simulink library "FUSI"  (R2024b)
settings: Solver=VariableStepAuto  StartTime=0.0  StopTime=10.0  RelTol=1e-3
libraries: simulink x1, FUSA_ACTMON x1, FUSA_FAULTVAIMAN x1, FUSA_SENSMON x1
settings Model: Creator=blatak  LastModifiedBy=jmbsp
settings ModelReferenceCC: EnableRefExpFcnMdlSchedulingChecks=on
settings RTWCC: GPUComputeCapability=3.5

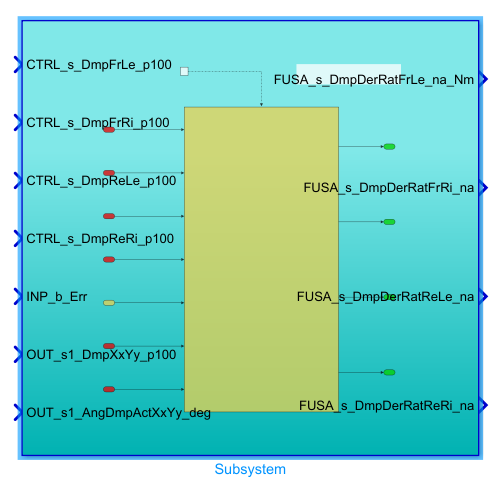
[thumbnail: Simulink's stored preview of the top-level diagram]
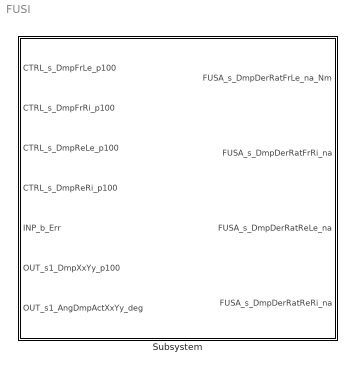
== system FUSI ==
  Subsystem : Subsystem

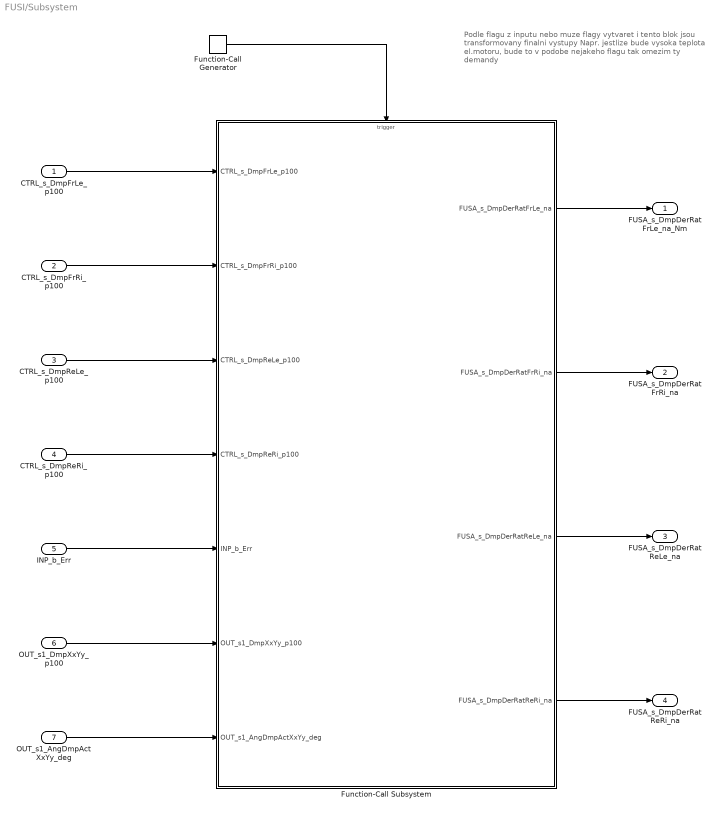
== system FUSI/Subsystem ==
  note: Podle flagu z inputu nebo muze flagy vytvaret i tento blok
      | jsou transformovany finalni vystupy
      | Napr. jestlize bude vysoka teplota el.motoru, bude to v podobe
      | nejakeho flagu tak omezim ty demandy
  CTRL_s_DmpFrLe_p100 : Inport
  CTRL_s_DmpFrRi_p100 : Inport  Port=2
  CTRL_s_DmpReLe_p100 : Inport  Port=3
  CTRL_s_DmpReRi_p100 : Inport  Port=4
  INP_b_Err : Inport  Port=5  OutDataTypeStr=Bus: INP_b_Err
  OUT_s1_DmpXxYy_p100 : Inport  Port=6
  OUT_s1_AngDmpActXxYy_deg : Inport  Port=7
  Function-Call Generator : simulink/Ports & Subsystems/Function-Call Generator  sample_time=0.005  numberOfIterations=1  DisallowWideOutput=off
  Function-Call Subsystem : Subsystem  TreatAsAtomicUnit=on
  FUSA_s_DmpDerRatFrLe_na_Nm : Outport
  FUSA_s_DmpDerRatFrRi_na : Outport  Port=2
  FUSA_s_DmpDerRatReLe_na : Outport  Port=3
  FUSA_s_DmpDerRatReRi_na : Outport  Port=4
  wires:
  Function-Call Generator/1 -> Function-Call Subsystem/Trigger
  CTRL_s_DmpFrLe_p100/1 -> Function-Call Subsystem/1(CTRL_s_DmpFrLe_p100)
  CTRL_s_DmpFrRi_p100/1 -> Function-Call Subsystem/2(CTRL_s_DmpFrRi_p100)
  CTRL_s_DmpReLe_p100/1 -> Function-Call Subsystem/3(CTRL_s_DmpReLe_p100)
  CTRL_s_DmpReRi_p100/1 -> Function-Call Subsystem/4(CTRL_s_DmpReRi_p100)
  Function-Call Subsystem/1(FUSA_s_DmpDerRatFrLe_na) -> FUSA_s_DmpDerRatFrLe_na_Nm/1
  INP_b_Err/1 -> Function-Call Subsystem/5(INP_b_Err)
  Function-Call Subsystem/2(FUSA_s_DmpDerRatFrRi_na) -> FUSA_s_DmpDerRatFrRi_na/1
  Function-Call Subsystem/3(FUSA_s_DmpDerRatReLe_na) -> FUSA_s_DmpDerRatReLe_na/1
  Function-Call Subsystem/4(FUSA_s_DmpDerRatReRi_na) -> FUSA_s_DmpDerRatReRi_na/1
  OUT_s1_DmpXxYy_p100/1 -> Function-Call Subsystem/6(OUT_s1_DmpXxYy_p100)
  OUT_s1_AngDmpActXxYy_deg/1 -> Function-Call Subsystem/7(OUT_s1_AngDmpActXxYy_deg)

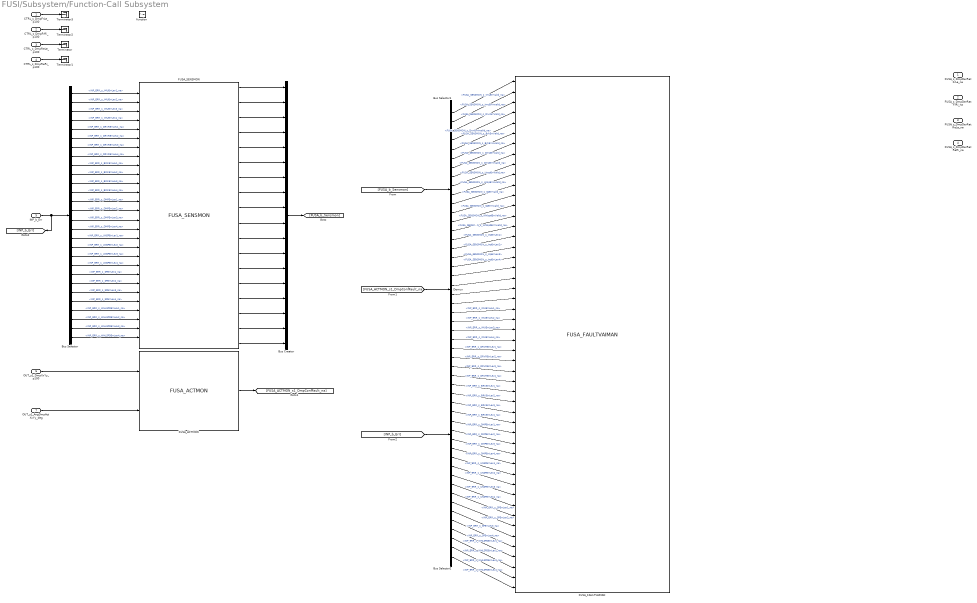
== system FUSI/Subsystem/Function-Call Subsystem ==
  CTRL_s_DmpFrLe_p100 : Inport
  CTRL_s_DmpFrRi_p100 : Inport  Port=2
  CTRL_s_DmpReLe_p100 : Inport  Port=3
  CTRL_s_DmpReRi_p100 : Inport  Port=4
  INP_b_Err : Inport  Port=5  OutDataTypeStr=Bus: INP_b_Err
  OUT_s1_DmpXxYy_p100 : Inport  Port=6
  OUT_s1_AngDmpActXxYy_deg : Inport  Port=7
  function : TriggerPort  TriggerType=function-call  VariantControl=(inherit)
  Bus Creator : BusCreator  Inputs=18  OutDataTypeStr=Bus: FUSA_b_Sensmon
      settings: InheritFromInputs=off
  Bus Selector : BusSelector  OutputSignals=INP_ERR_s_IMUErrLev1_na,INP_ERR_s_IMUErrLev2_na,INP_ERR_s_IMUErrLev3_na,INP_ERR_s_IMUErrLev4_na,INP_ERR_s_DRVRErrLev1_na,INP_ERR_s_DRVRErrLev2_na,INP_ERR_s_DRVRErrLev3_na,INP_ERR_s_DRVRErrLev4_na,INP_ERR_s_BRKErrLev1_na,INP_ERR_s_BRKErrLev2_na,INP_ERR_s_BRKErrLev3_na,INP_ERR_s_BRKErrLev4_na,INP_ERR_s_DMPErrLev1_na,INP_ERR_s_DMPErrLev2_na,INP_ERR_s_DMPErrLev3_na,INP_ERR_s_DMPErrLev4_na,INP_ERR_s_UNSPErrLev1_na,INP_ERR_s_UNSPErrLev2_na,INP_ERR_s_UNSPErrLev3_na,INP_ERR_s_UNSPErrLev4_na,INP_ERR_s_SPErrLev1_na,INP_ERR_s_SPErrLev2_na,INP_ERR_s_SPErrLev3_na,INP_ERR_s_SPErrLev4_na,INP_ERR_s_WHLSPDErrLev1_na,INP_ERR_s_WHLSPDErrLev2_na,INP_ERR_s_WHLSPDErrLev3_na,INP_ERR_s_WHLSPDErrLev4_na
  Bus Selector1 : BusSelector  OutputSignals=FUSA_SENSMON_s_ImuErrValid_na,FUSA_SENSMON_s_ImuErrInvalid_na,FUSA_SENSMON_s_DrvrErrValid_na,FUSA_SENSMON_s_DrvrErrInvalid_na,FUSA_SENSMON_s_BrkErrValid_na,FUSA_SENSMON_s_BrkErrInvalid_na,FUSA_SENSMON_s_DmpErrValid_na,FUSA_SENSMON_s_DmpErrInvalid_na,FUSA_SENSMON_s_UnspErrValid_na,FUSA_SENSMON_s_UnspErrInvalid_na,FUSA_SENSMON_s_SpErrValid_na,FUSA_SENSMON_s_SpErrInvalid_na,FUSA_SENSMON_s_WhlspdErrValid_na,FUSA_SENSMON_s_WhlspdErrInvalid_na,FUSA_SENSMON_s_InpErrLev1,FUSA_SENSMON_s_InpErrLev2,FUSA_SENSMON_s_InpErrLev3,FUSA_SENSMON_s_InpErrLev4
  Bus Selector2 : BusSelector  OutputSignals=INP_ERR_s_IMUErrLev1_na,INP_ERR_s_IMUErrLev2_na,INP_ERR_s_IMUErrLev3_na,INP_ERR_s_IMUErrLev4_na,INP_ERR_s_DRVRErrLev1_na,INP_ERR_s_DRVRErrLev2_na,INP_ERR_s_DRVRErrLev3_na,INP_ERR_s_DRVRErrLev4_na,INP_ERR_s_BRKErrLev1_na,INP_ERR_s_BRKErrLev2_na,INP_ERR_s_BRKErrLev3_na,INP_ERR_s_BRKErrLev4_na,INP_ERR_s_DMPErrLev1_na,INP_ERR_s_DMPErrLev2_na,INP_ERR_s_DMPErrLev3_na,INP_ERR_s_DMPErrLev4_na,INP_ERR_s_UNSPErrLev1_na,INP_ERR_s_UNSPErrLev2_na,INP_ERR_s_UNSPErrLev3_na,INP_ERR_s_UNSPErrLev4_na,INP_ERR_s_SPErrLev1_na,INP_ERR_s_SPErrLev2_na,INP_ERR_s_SPErrLev3_na,INP_ERR_s_SPErrLev4_na,INP_ERR_s_WHLSPDErrLev1_na,INP_ERR_s_WHLSPDErrLev2_na,INP_ERR_s_WHLSPDErrLev3_na,INP_ERR_s_WHLSPDErrLev4_na
  Demux : Demux
  FUSA_ACTMON : FUSA_ACTMON/FUSA_ACTMON  SystemSampleTime=-1  VariantActivationTime=update diagram  AllowFlexibleInterface=on  Latency=0  AutoFrameSizeCalculation=off
  FUSA_FAULTVAIMAN : FUSA_FAULTVAIMAN/FUSA_FAULTVAIMAN  SystemSampleTime=-1  VariantActivationTime=update diagram  AllowFlexibleInterface=on  Latency=0  AutoFrameSizeCalculation=off
  FUSA_SENSMON : FUSA_SENSMON/FUSA_SENSMON  SystemSampleTime=-1  VariantActivationTime=update diagram  AllowFlexibleInterface=on  Latency=0  AutoFrameSizeCalculation=off
  Terminator{,1..3} (4 alike) : Terminator
  FUSA_s_DmpDerRatFrLe_na : Outport
  FUSA_s_DmpDerRatFrRi_na : Outport  Port=2
  FUSA_s_DmpDerRatReLe_na : Outport  Port=3
  FUSA_s_DmpDerRatReRi_na : Outport  Port=4
  wires:
  INP_b_Err/1 -> [INP_b_Err], Bus Selector/1
  OUT_s1_DmpXxYy_p100/1 -> FUSA_ACTMON/1
  OUT_s1_AngDmpActXxYy_deg/1 -> FUSA_ACTMON/2
  Bus Selector/23 -> FUSA_SENSMON/23  "<INP_ERR_s_SPErrLev3_na>"
  Bus Selector/24 -> FUSA_SENSMON/24  "<INP_ERR_s_SPErrLev4_na>"
  Bus Selector/22 -> FUSA_SENSMON/22  "<INP_ERR_s_SPErrLev2_na>"
  Bus Selector/25 -> FUSA_SENSMON/25  "<INP_ERR_s_WHLSPDErrLev1_na>"
  Bus Selector/21 -> FUSA_SENSMON/21  "<INP_ERR_s_SPErrLev1_na>"
  Bus Selector/26 -> FUSA_SENSMON/26  "<INP_ERR_s_WHLSPDErrLev2_na>"
  Bus Selector/20 -> FUSA_SENSMON/20  "<INP_ERR_s_UNSPErrLev4_na>"
  Bus Selector/27 -> FUSA_SENSMON/27  "<INP_ERR_s_WHLSPDErrLev3_na>"
  Bus Selector/19 -> FUSA_SENSMON/19  "<INP_ERR_s_UNSPErrLev3_na>"
  Bus Selector/28 -> FUSA_SENSMON/28  "<INP_ERR_s_WHLSPDErrLev4_na>"
  Bus Selector/18 -> FUSA_SENSMON/18  "<INP_ERR_s_UNSPErrLev2_na>"
  Bus Selector/17 -> FUSA_SENSMON/17  "<INP_ERR_s_UNSPErrLev1_na>"
  Bus Selector/16 -> FUSA_SENSMON/16  "<INP_ERR_s_DMPErrLev4_na>"
  Bus Selector/15 -> FUSA_SENSMON/15  "<INP_ERR_s_DMPErrLev3_na>"
  Bus Selector/14 -> FUSA_SENSMON/14  "<INP_ERR_s_DMPErrLev2_na>"
  Bus Selector/13 -> FUSA_SENSMON/13  "<INP_ERR_s_DMPErrLev1_na>"
  Bus Selector/12 -> FUSA_SENSMON/12  "<INP_ERR_s_BRKErrLev4_na>"
  Bus Selector/11 -> FUSA_SENSMON/11  "<INP_ERR_s_BRKErrLev3_na>"
  Bus Selector/10 -> FUSA_SENSMON/10  "<INP_ERR_s_BRKErrLev2_na>"
  Bus Selector/9 -> FUSA_SENSMON/9  "<INP_ERR_s_BRKErrLev1_na>"
  Bus Selector/8 -> FUSA_SENSMON/8  "<INP_ERR_s_DRVRErrLev4_na>"
  Bus Selector/7 -> FUSA_SENSMON/7  "<INP_ERR_s_DRVRErrLev3_na>"
  Bus Selector/6 -> FUSA_SENSMON/6  "<INP_ERR_s_DRVRErrLev2_na>"
  Bus Selector/5 -> FUSA_SENSMON/5  "<INP_ERR_s_DRVRErrLev1_na>"
  Bus Selector/4 -> FUSA_SENSMON/4  "<INP_ERR_s_IMUErrLev4_na>"
  Bus Selector/3 -> FUSA_SENSMON/3  "<INP_ERR_s_IMUErrLev3_na>"
  Bus Selector/2 -> FUSA_SENSMON/2  "<INP_ERR_s_IMUErrLev2_na>"
  Bus Selector/1 -> FUSA_SENSMON/1  "<INP_ERR_s_IMUErrLev1_na>"
  FUSA_SENSMON/1 -> Bus Creator/1
  FUSA_SENSMON/2 -> Bus Creator/2
  FUSA_SENSMON/3 -> Bus Creator/3
  FUSA_SENSMON/4 -> Bus Creator/4
  FUSA_SENSMON/5 -> Bus Creator/5
  FUSA_SENSMON/6 -> Bus Creator/6
  FUSA_SENSMON/7 -> Bus Creator/7
  FUSA_SENSMON/8 -> Bus Creator/8
  FUSA_SENSMON/9 -> Bus Creator/9
  FUSA_SENSMON/10 -> Bus Creator/10
  FUSA_SENSMON/11 -> Bus Creator/11
  FUSA_SENSMON/12 -> Bus Creator/12
  FUSA_SENSMON/13 -> Bus Creator/13
  FUSA_SENSMON/14 -> Bus Creator/14
  FUSA_SENSMON/15 -> Bus Creator/15
  FUSA_SENSMON/16 -> Bus Creator/16
  FUSA_SENSMON/17 -> Bus Creator/17
  FUSA_SENSMON/18 -> Bus Creator/18
  Bus Creator/1 -> [FUSA_b_Sensmon]
  CTRL_s_DmpReLe_p100/1 -> Terminator/1
  CTRL_s_DmpReRi_p100/1 -> Terminator1/1
  CTRL_s_DmpFrRi_p100/1 -> Terminator2/1
  CTRL_s_DmpFrLe_p100/1 -> Terminator3/1
  FUSA_ACTMON/1 -> [FUSA_ACTMON_s1_DmpConfFault_na]
  [FUSA_ACTMON_s1_DmpConfFault_na] -> Demux/1
  [FUSA_b_Sensmon] -> Bus Selector1/1
  Bus Selector1/1 -> FUSA_FAULTVAIMAN/1  "<FUSA_SENSMON_s_ImuErrValid_na>"
  Bus Selector1/2 -> FUSA_FAULTVAIMAN/2  "<FUSA_SENSMON_s_ImuErrInvalid_na>"
  Bus Selector1/3 -> FUSA_FAULTVAIMAN/3  "<FUSA_SENSMON_s_DrvrErrValid_na>"
  Bus Selector1/4 -> FUSA_FAULTVAIMAN/4  "<FUSA_SENSMON_s_DrvrErrInvalid_na>"
  Bus Selector1/5 -> FUSA_FAULTVAIMAN/5  "<FUSA_SENSMON_s_BrkErrValid_na>"
  Bus Selector1/6 -> FUSA_FAULTVAIMAN/6  "<FUSA_SENSMON_s_BrkErrInvalid_na>"
  Bus Selector1/7 -> FUSA_FAULTVAIMAN/7  "<FUSA_SENSMON_s_DmpErrValid_na>"
  Bus Selector1/8 -> FUSA_FAULTVAIMAN/8  "<FUSA_SENSMON_s_DmpErrInvalid_na>"
  Bus Selector1/9 -> FUSA_FAULTVAIMAN/9  "<FUSA_SENSMON_s_UnspErrValid_na>"
  Bus Selector1/10 -> FUSA_FAULTVAIMAN/10  "<FUSA_SENSMON_s_UnspErrInvalid_na>"
  Bus Selector1/11 -> FUSA_FAULTVAIMAN/11  "<FUSA_SENSMON_s_SpErrValid_na>"
  Bus Selector1/12 -> FUSA_FAULTVAIMAN/12  "<FUSA_SENSMON_s_SpErrInvalid_na>"
  Bus Selector1/13 -> FUSA_FAULTVAIMAN/13  "<FUSA_SENSMON_s_WhlspdErrValid_na>"
  Bus Selector1/14 -> FUSA_FAULTVAIMAN/14  "<FUSA_SENSMON_s_WhlspdErrInvalid_na>"
  Bus Selector1/15 -> FUSA_FAULTVAIMAN/15  "<FUSA_SENSMON_s_InpErrLev1>"
  Bus Selector1/16 -> FUSA_FAULTVAIMAN/16  "<FUSA_SENSMON_s_InpErrLev2>"
  Bus Selector1/17 -> FUSA_FAULTVAIMAN/17  "<FUSA_SENSMON_s_InpErrLev3>"
  Bus Selector1/18 -> FUSA_FAULTVAIMAN/18  "<FUSA_SENSMON_s_InpErrLev4>"
  Demux/1 -> FUSA_FAULTVAIMAN/19
  Demux/2 -> FUSA_FAULTVAIMAN/20
  Demux/3 -> FUSA_FAULTVAIMAN/21
  Demux/4 -> FUSA_FAULTVAIMAN/22
  [INP_b_Err] -> Bus Selector2/1
  Bus Selector2/3 -> FUSA_FAULTVAIMAN/25  "<INP_ERR_s_IMUErrLev3_na>"
  Bus Selector2/4 -> FUSA_FAULTVAIMAN/26  "<INP_ERR_s_IMUErrLev4_na>"
  Bus Selector2/2 -> FUSA_FAULTVAIMAN/24  "<INP_ERR_s_IMUErrLev2_na>"
  Bus Selector2/5 -> FUSA_FAULTVAIMAN/27  "<INP_ERR_s_DRVRErrLev1_na>"
  Bus Selector2/1 -> FUSA_FAULTVAIMAN/23  "<INP_ERR_s_IMUErrLev1_na>"
  Bus Selector2/6 -> FUSA_FAULTVAIMAN/28  "<INP_ERR_s_DRVRErrLev2_na>"
  Bus Selector2/7 -> FUSA_FAULTVAIMAN/29  "<INP_ERR_s_DRVRErrLev3_na>"
  Bus Selector2/8 -> FUSA_FAULTVAIMAN/30  "<INP_ERR_s_DRVRErrLev4_na>"
  Bus Selector2/9 -> FUSA_FAULTVAIMAN/31  "<INP_ERR_s_BRKErrLev1_na>"
  Bus Selector2/10 -> FUSA_FAULTVAIMAN/32  "<INP_ERR_s_BRKErrLev2_na>"
  Bus Selector2/11 -> FUSA_FAULTVAIMAN/33  "<INP_ERR_s_BRKErrLev3_na>"
  Bus Selector2/12 -> FUSA_FAULTVAIMAN/34  "<INP_ERR_s_BRKErrLev4_na>"
  Bus Selector2/13 -> FUSA_FAULTVAIMAN/35  "<INP_ERR_s_DMPErrLev1_na>"
  Bus Selector2/14 -> FUSA_FAULTVAIMAN/36  "<INP_ERR_s_DMPErrLev2_na>"
  Bus Selector2/15 -> FUSA_FAULTVAIMAN/37  "<INP_ERR_s_DMPErrLev3_na>"
  Bus Selector2/16 -> FUSA_FAULTVAIMAN/38  "<INP_ERR_s_DMPErrLev4_na>"
  Bus Selector2/17 -> FUSA_FAULTVAIMAN/39  "<INP_ERR_s_UNSPErrLev1_na>"
  Bus Selector2/18 -> FUSA_FAULTVAIMAN/40  "<INP_ERR_s_UNSPErrLev2_na>"
  Bus Selector2/19 -> FUSA_FAULTVAIMAN/41  "<INP_ERR_s_UNSPErrLev3_na>"
  Bus Selector2/20 -> FUSA_FAULTVAIMAN/42  "<INP_ERR_s_UNSPErrLev4_na>"
  Bus Selector2/21 -> FUSA_FAULTVAIMAN/43  "<INP_ERR_s_SPErrLev1_na>"
  Bus Selector2/22 -> FUSA_FAULTVAIMAN/44  "<INP_ERR_s_SPErrLev2_na>"
  Bus Selector2/23 -> FUSA_FAULTVAIMAN/45  "<INP_ERR_s_SPErrLev3_na>"
  Bus Selector2/24 -> FUSA_FAULTVAIMAN/46  "<INP_ERR_s_SPErrLev4_na>"
  Bus Selector2/25 -> FUSA_FAULTVAIMAN/47  "<INP_ERR_s_WHLSPDErrLev1_na>"
  Bus Selector2/26 -> FUSA_FAULTVAIMAN/48  "<INP_ERR_s_WHLSPDErrLev2_na>"
  Bus Selector2/27 -> FUSA_FAULTVAIMAN/49  "<INP_ERR_s_WHLSPDErrLev3_na>"
  Bus Selector2/28 -> FUSA_FAULTVAIMAN/50  "<INP_ERR_s_WHLSPDErrLev4_na>"
